simulink model "sampleModel1561_4"  (R2023a)
settings: Solver=VariableStepAuto  StartTime=0.0  StopTime=10.0  RelTol=1e-3
libraries: hdlsllib x5, simulink x2
settings Model: Creator=user1  LastModifiedBy=user1

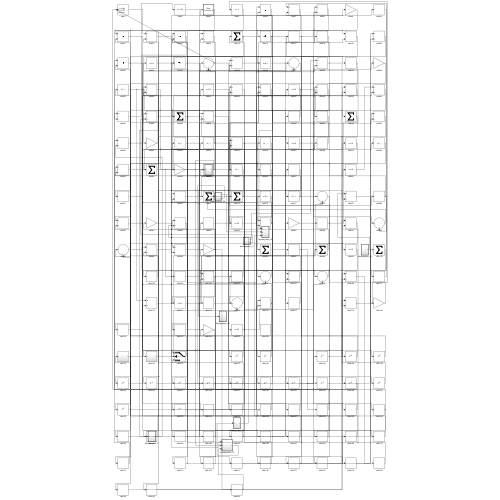
[thumbnail: Simulink's stored preview of the top-level diagram]
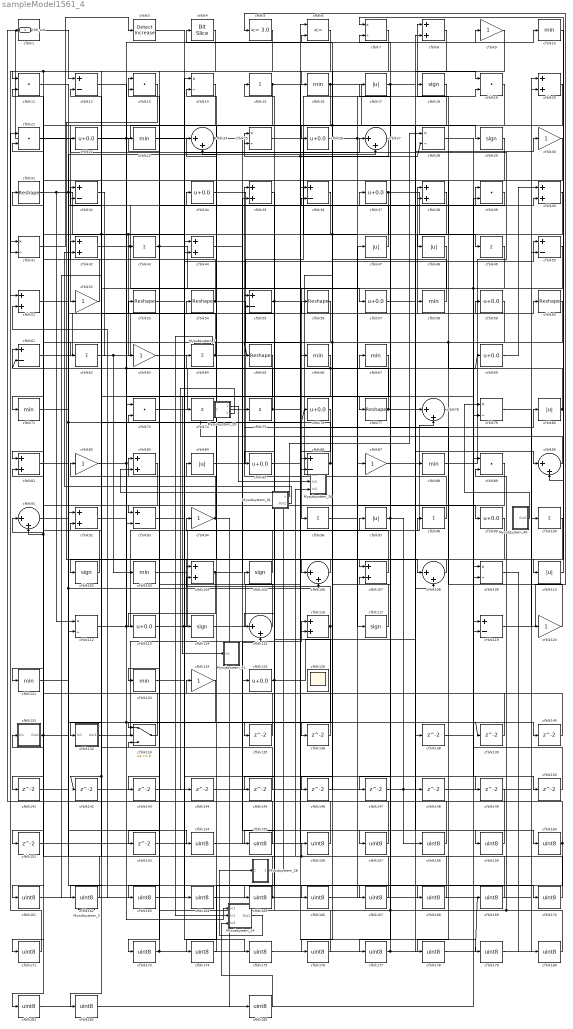
== system sampleModel1561_4 ==
  Mysubsystem_14 : Subsystem  TreatAsAtomicUnit=on  RTWFcnName=Mysubsystem_14
      settings: RTWFcnNameOpts=User specified  RTWFileNameOpts=Use function name
  Mysubsystem_26 : Subsystem  TreatAsAtomicUnit=on  RTWFcnName=Mysubsystem_26
      settings: RTWFcnNameOpts=User specified  RTWFileNameOpts=Use function name
  Mysubsystem_28 : Subsystem  TreatAsAtomicUnit=on  RTWFcnName=Mysubsystem_28
      settings: RTWFcnNameOpts=User specified  RTWFileNameOpts=Use function name
  Mysubsystem_29 : Subsystem  TreatAsAtomicUnit=on  RTWFcnName=Mysubsystem_29
      settings: RTWFcnNameOpts=User specified  RTWFileNameOpts=Use function name
  Mysubsystem_3 : Subsystem  TreatAsAtomicUnit=on  RTWFcnName=Mysubsystem_3
      settings: RTWFcnNameOpts=User specified  RTWFileNameOpts=Use function name
  Mysubsystem_31 : Subsystem  TreatAsAtomicUnit=on  RTWFcnName=Mysubsystem_31
      settings: RTWFcnNameOpts=User specified  RTWFileNameOpts=Use function name
  Mysubsystem_40 : Subsystem  TreatAsAtomicUnit=on  RTWFcnName=Mysubsystem_40
      settings: RTWFcnNameOpts=User specified  RTWFileNameOpts=Use function name
  Mysubsystem_41 : Subsystem  TreatAsAtomicUnit=on  RTWFcnName=Mysubsystem_41
      settings: RTWFcnNameOpts=User specified  RTWFileNameOpts=Use function name
  Mysubsystem_7 : Subsystem  TreatAsAtomicUnit=on  RTWFcnName=Mysubsystem_7
      settings: RTWFcnNameOpts=User specified  RTWFileNameOpts=Use function name
  cfblk1 : simulink/Logic and Bit Operations/Bit Set  iBit=0
      settings: LibrarySourceBlock=|
      | hdlsllib/Logic and Bit
      | Operations/Bit Set
  cfblk{10,16,23,58,66..67,71,88,103,121,123} (11 alike) : MinMax  OutDataTypeStr=uint8
  cfblk{15,43,49,62,64,74..75,96,98,100} (10 alike) : Sum  Inputs=+  OutDataTypeStr=uint8
  cfblk{18,29,102,105,114,117} (6 alike) : Signum
  cfblk{8,20,35,38,40,42,44,51,81,83,92,104,107,116} (14 alike) : Sum  OutDataTypeStr=uint8
  cfblk{24,27,78,90..91,106,108,115} (8 alike) : Sum  Inputs=|++  OutDataTypeStr=uint8
  cfblk{7,14,25,28,41,79,109,112} (8 alike) : Product  Inputs=*/  OutDataTypeStr=uint8  RndMeth=Zero  SaturateOnIntegerOverflow=on
  cfblk{11,13,19,21,39,73,89} (7 alike) : DotProduct  OutDataTypeStr=uint8
  cfblk{17,47..48,80,84,97,110} (7 alike) : Abs  OutDataTypeStr=uint8  SaturateOnIntegerOverflow=off
  cfblk{22,26,34,37,57,59,69,76,85,99,113,125} (12 alike) : Bias  Bias=0.0  SaturateOnIntegerOverflow=off
  cfblk{12,32,36,50,55,61,86,93,119} (9 alike) : Sum  Inputs=+-  OutDataTypeStr=uint8
  cfblk{9,30,52,63,82,87,94,120,124} (9 alike) : Gain  OutDataTypeStr=uint8
  cfblk126 : Scope
      settings: Floating=on
  cfblk131 : Subsystem
      settings: LibrarySourceBlock=|
      | hdlsllib/Ports &
      | Subsystems/Subsystem
  cfblk132 : Subsystem
      settings: LibrarySourceBlock=|
      | hdlsllib/Ports &
      | Subsystems/Subsystem
  cfblk133 : Switch  OutDataTypeStr=uint8  SaturateOnIntegerOverflow=off  InputSameDT=off
  cfblk{135..136,138..151,153} (17 alike) : Delay  SampleTime=1
  cfblk{154..171,173..182,185} (29 alike) : DataTypeConversion  OutDataTypeStr=uint8  SaturateOnIntegerOverflow=off  RndMeth=Floor
  cfblk3 : simulink/Logic and Bit Operations/Detect Increase  vinit=0.0  OutDataTypeStr=uint8
      settings: LibrarySourceBlock=|
      | hdlsllib/Logic and Bit
      | Operations/Detect
      | Increase
  cfblk{31,53..54,56,60,65,77} (7 alike) : Reshape
  cfblk4 : hdlsllib/Logic and Bit Operations/Bit Slice  lidx=7  ridx=0
  cfblk5 : hdlsllib/Logic and Bit Operations/Compare To Constant  relop=<=  const=3.0  OutDataTypeStr=uint8
  cfblk6 : RelationalOperator  Operator=<=  OutDataTypeStr=boolean  InputSameDT=off
  Hdl_out : Outport  OutDataTypeStr=uint8
  wires:
  cfblk9/1 -> cfblk16/1
  cfblk89/1 -> cfblk93/1
  cfblk15/1 -> cfblk52/1, cfblk159/1
  cfblk37/1 -> Mysubsystem_26/1(In1), Mysubsystem_3/1(In1), cfblk151/1, cfblk49/1
  cfblk48/1 -> cfblk96/1
  cfblk34/1 -> cfblk57/1
  cfblk13/1 -> cfblk108/1
  cfblk88/1 -> cfblk25/1
  cfblk47/1 -> cfblk13/1
  cfblk97/1 -> cfblk148/1, cfblk158/1, cfblk147/1
  cfblk98/1 -> cfblk35/1
  cfblk66/1 -> Mysubsystem_41/1(In1), cfblk61/2
  cfblk61/1 -> cfblk38/1
  cfblk41/1 -> cfblk3/1
  cfblk58/1 -> cfblk4/1
  cfblk105/1 -> cfblk94/1
  cfblk17/1 -> cfblk77/1, cfblk19/1
  cfblk113/1 -> cfblk97/1, cfblk149/1
  cfblk64/1 -> cfblk56/1, cfblk32/1
  cfblk109/1 -> cfblk180/1
  cfblk87/1 -> cfblk160/1
  cfblk110/1 -> cfblk7/1
  cfblk62/1 -> cfblk54/1, cfblk103/1
  cfblk59/1 -> cfblk106/1, cfblk141/1
  cfblk65/1 -> cfblk142/1, cfblk182/1
  cfblk29/1 -> cfblk48/1
  cfblk99/1 -> cfblk114/1
  cfblk31/1 -> cfblk43/1, cfblk74/1, cfblk135/1, cfblk112/1
  cfblk86/1 -> cfblk32/2, cfblk136/1
  cfblk119/1 -> cfblk5/1
  cfblk69/1 -> cfblk40/1
  cfblk103/1 -> cfblk35/2
  cfblk112/1 -> cfblk69/1, cfblk55/2, cfblk78/2
  cfblk114/1 -> cfblk80/1
  cfblk74/1 -> cfblk8/1
  cfblk84/1 -> cfblk39/1
  cfblk79/1 -> cfblk120/1
  cfblk94/1 -> cfblk82/1, cfblk185/1
  cfblk36/1 -> cfblk63/1
  cfblk18/1 -> cfblk121/1
  cfblk76/1 -> cfblk86/1
  cfblk133/1 -> cfblk91/1, cfblk91/2
  cfblk104/1 -> cfblk113/1, cfblk98/1
  cfblk120/1 -> cfblk75/1
  cfblk115/1 -> cfblk83/1
  cfblk93/1 -> cfblk27/1
  cfblk80/1 -> cfblk18/1, cfblk90/2
  cfblk106/1 -> cfblk102/1
  cfblk116/1 -> cfblk104/2, cfblk163/1
  cfblk10/1 -> cfblk110/1
  cfblk25/1 -> cfblk117/1
  cfblk22/1 -> Mysubsystem_14/1(In1), cfblk29/1
  cfblk132/1(Out1) -> cfblk116/1
  cfblk107/1 -> cfblk64/1
  cfblk67/1 -> cfblk115/1
  cfblk124/1 -> cfblk173/1
  cfblk5/1 -> cfblk132/1(In1)
  cfblk92/1 -> cfblk167/1
  cfblk39/1 -> cfblk36/2
  cfblk63/1 -> cfblk50/1
  cfblk38/1 -> cfblk123/1
  cfblk75/1 -> cfblk53/1, cfblk179/1
  cfblk60/1 -> cfblk65/1, cfblk178/1
  cfblk54/1 -> cfblk66/1, cfblk11/2
  cfblk121/1 -> cfblk27/2
  cfblk20/1 -> cfblk177/1
  cfblk7/1 -> cfblk11/1
  cfblk43/1 -> cfblk125/1, cfblk153/1
  cfblk125/1 -> cfblk15/1, cfblk8/2
  cfblk42/1 -> cfblk86/2, cfblk37/1
  cfblk26/1 -> cfblk99/1, cfblk19/2
  cfblk96/1 -> cfblk58/1
  cfblk8/1 -> cfblk26/1
  cfblk77/1 -> cfblk30/1, cfblk55/1
  cfblk71/1 -> cfblk34/1
  cfblk19/1 -> cfblk104/1, cfblk146/1
  cfblk55/1 -> cfblk38/2, cfblk145/1
  cfblk85/1 -> cfblk10/1, cfblk28/2
  cfblk27/1 -> cfblk25/2
  cfblk81/1 -> cfblk76/1, cfblk60/1
  cfblk16/1 -> cfblk88/1, cfblk133/1
  cfblk100/1 -> cfblk165/1
  cfblk108/1 -> cfblk107/1
  cfblk117/1 -> cfblk22/1
  cfblk35/1 -> cfblk85/1
  cfblk50/1 -> cfblk119/2, cfblk62/1
  cfblk52/1 -> cfblk42/1
  cfblk82/1 -> cfblk93/2, cfblk9/1
  cfblk91/1 -> cfblk59/1
  cfblk123/1 -> cfblk44/1
  cfblk6/1 -> cfblk81/1, cfblk41/2
  cfblk11/1 -> cfblk133/2, cfblk139/1, cfblk106/2
  cfblk30/1 -> cfblk71/1
  cfblk12/1 -> cfblk79/2
  cfblk57/1 -> cfblk90/1
  cfblk73/1 -> cfblk67/1
  cfblk3/1 -> cfblk44/2
  cfblk131/1(Out1) -> cfblk40/2, cfblk181/1
  cfblk1/1 -> cfblk12/1
  cfblk102/1 -> cfblk61/1
  cfblk135/1 -> cfblk13/2
  cfblk136/1 -> cfblk73/1
  cfblk138/1 -> cfblk39/2
  cfblk139/1 -> cfblk107/2
  cfblk44/1 -> cfblk140/1
  cfblk140/1 -> cfblk81/2
  cfblk141/1 -> cfblk112/2
  cfblk142/1 -> cfblk78/1
  cfblk4/1 -> cfblk143/1
  cfblk144/1 -> cfblk36/1
  cfblk145/1 -> cfblk12/2
  cfblk146/1 -> cfblk6/2
  cfblk147/1 -> cfblk108/2
  cfblk148/1 -> cfblk50/2
  cfblk149/1 -> cfblk1/1
  cfblk28/1 -> cfblk150/1
  cfblk150/1 -> cfblk119/1
  cfblk151/1 -> cfblk116/2
  cfblk153/1 -> cfblk115/2
  cfblk21/1 -> cfblk154/1
  cfblk154/1 -> cfblk6/1
  cfblk49/1 -> cfblk155/1
  cfblk155/1 -> cfblk21/1
  cfblk156/1 -> cfblk21/2
  cfblk24/1 -> cfblk157/1, Hdl_out/1
  cfblk157/1 -> cfblk41/1
  cfblk158/1 -> cfblk24/1
  cfblk159/1 -> cfblk24/2
  cfblk160/1 -> cfblk133/3, cfblk174/1
  cfblk56/1 -> cfblk161/1
  cfblk161/1 -> cfblk87/1
  cfblk14/1 -> cfblk162/1
  cfblk162/1 -> cfblk31/1
  cfblk163/1 -> cfblk14/1
  cfblk143/1 -> cfblk164/1
  cfblk164/1 -> cfblk14/2
  cfblk165/1 -> cfblk131/1(In1), cfblk47/1
  cfblk53/1 -> cfblk166/1
  cfblk166/1 -> cfblk100/1
  cfblk167/1 -> Mysubsystem_26/3(In3), cfblk156/1
  cfblk78/1 -> cfblk168/1
  cfblk168/1 -> cfblk92/1
  cfblk169/1 -> cfblk92/2
  cfblk51/1 -> cfblk170/1
  cfblk170/1 -> cfblk84/1
  cfblk83/1 -> cfblk171/1
  cfblk171/1 -> cfblk51/1
  cfblk173/1 -> cfblk169/1, cfblk73/2
  cfblk174/1 -> cfblk124/1
  cfblk23/1 -> cfblk175/1
  cfblk175/1 -> cfblk89/1
  cfblk40/1 -> cfblk176/1
  cfblk176/1 -> cfblk23/1
  cfblk177/1 -> cfblk138/1, cfblk7/2
  cfblk178/1 -> cfblk20/1
  cfblk179/1 -> cfblk20/2
  cfblk180/1 -> cfblk17/1, cfblk105/1, cfblk89/2
  cfblk181/1 -> cfblk109/1
  cfblk182/1 -> cfblk109/2
  Mysubsystem_3/1(Out1) -> cfblk51/2
  cfblk32/1 -> Mysubsystem_7/1(u)
  Mysubsystem_7/1(Out1) -> Mysubsystem_14/2(In2)
  cfblk185/1 -> Mysubsystem_14/3(In3)
  Mysubsystem_14/1(Out1) -> Mysubsystem_28/1(In1)
  Mysubsystem_28/1(Out1) -> cfblk83/2
  cfblk90/1 -> Mysubsystem_29/1(In1)
  Mysubsystem_29/1(Out1) -> Mysubsystem_26/2(In2)
  Mysubsystem_29/2(Out2) -> cfblk144/1
  Mysubsystem_31/1(y) -> cfblk28/1
  Mysubsystem_31/2(Out2) -> cfblk42/2
  Mysubsystem_40/1(Out1) -> cfblk79/1

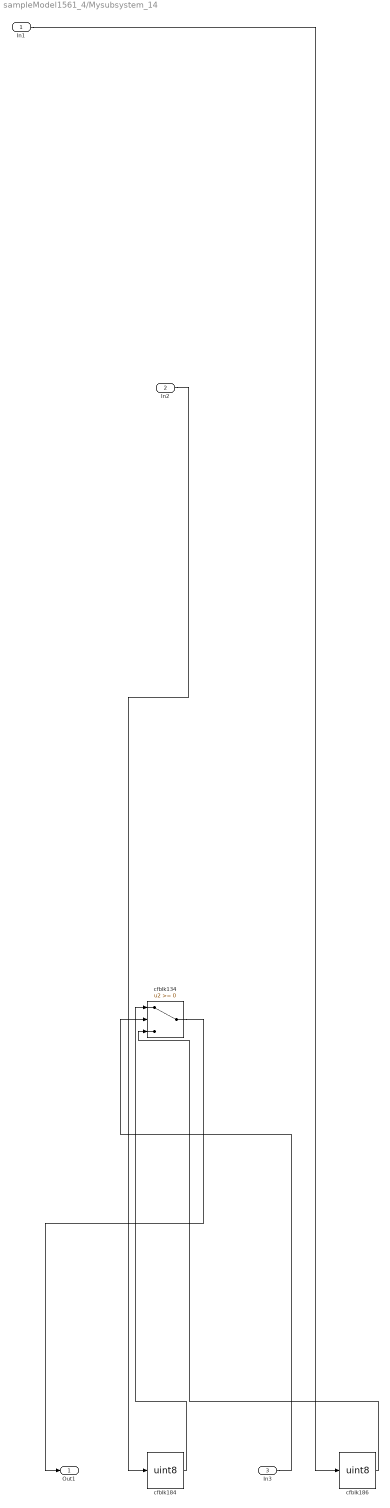
== system sampleModel1561_4/Mysubsystem_14 ==
  In1 : Inport
  In2 : Inport  Port=2
  In3 : Inport  Port=3
  cfblk134 : Switch  SaturateOnIntegerOverflow=off  InputSameDT=off
  cfblk184 : DataTypeConversion  OutDataTypeStr=uint8  SaturateOnIntegerOverflow=off  RndMeth=Floor
  cfblk186 : DataTypeConversion  OutDataTypeStr=uint8  SaturateOnIntegerOverflow=off  RndMeth=Floor
  Out1 : Outport
  wires:
  cfblk134/1 -> Out1/1
  cfblk186/1 -> cfblk134/3
  cfblk184/1 -> cfblk134/1
  In2/1 -> cfblk184/1
  In1/1 -> cfblk186/1
  In3/1 -> cfblk134/2

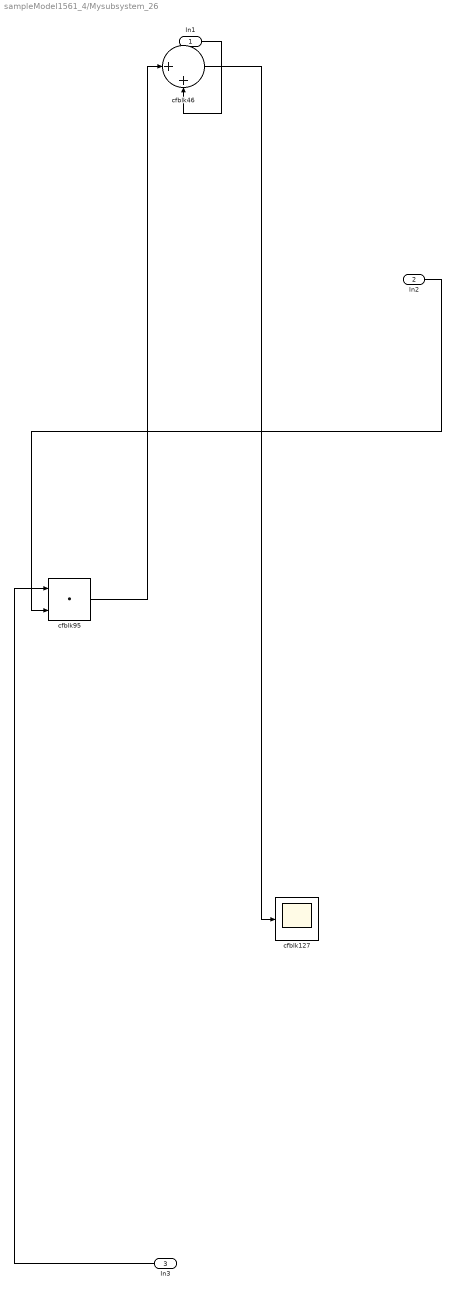
== system sampleModel1561_4/Mysubsystem_26 ==
  In1 : Inport
  In2 : Inport  Port=2
  In3 : Inport  Port=3
  cfblk127 : Scope
  cfblk46 : Sum  Inputs=|++
  cfblk95 : DotProduct  OutDataTypeStr=Inherit: Inherit via internal rule
  wires:
  cfblk95/1 -> cfblk46/1
  In1/1 -> cfblk46/2
  cfblk46/1 -> cfblk127/1
  In2/1 -> cfblk95/2
  In3/1 -> cfblk95/1

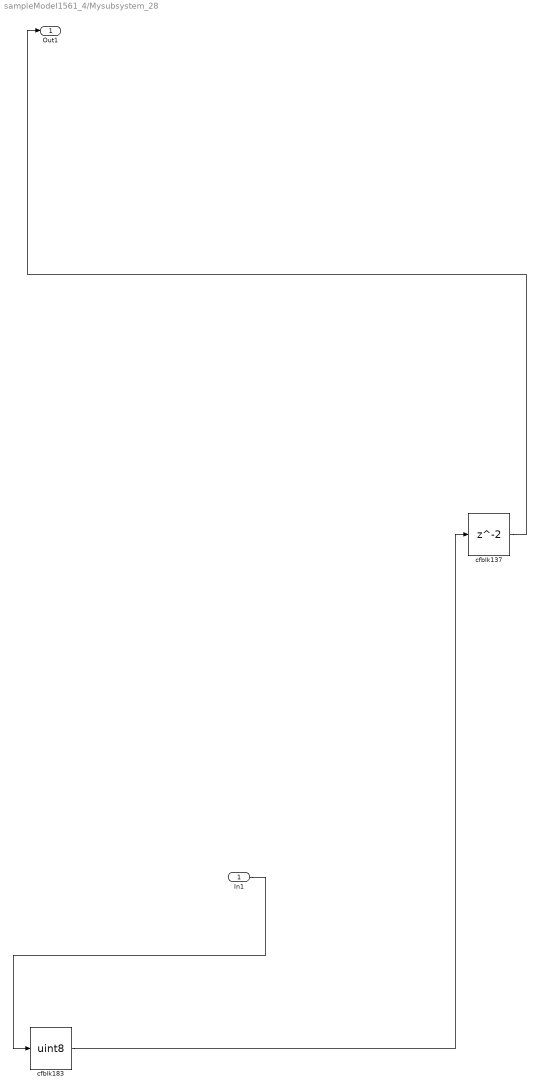
== system sampleModel1561_4/Mysubsystem_28 ==
  In1 : Inport
  cfblk137 : Delay  SampleTime=1
  cfblk183 : DataTypeConversion  OutDataTypeStr=uint8  SaturateOnIntegerOverflow=off  RndMeth=Floor
  Out1 : Outport
  wires:
  cfblk183/1 -> cfblk137/1
  cfblk137/1 -> Out1/1
  In1/1 -> cfblk183/1

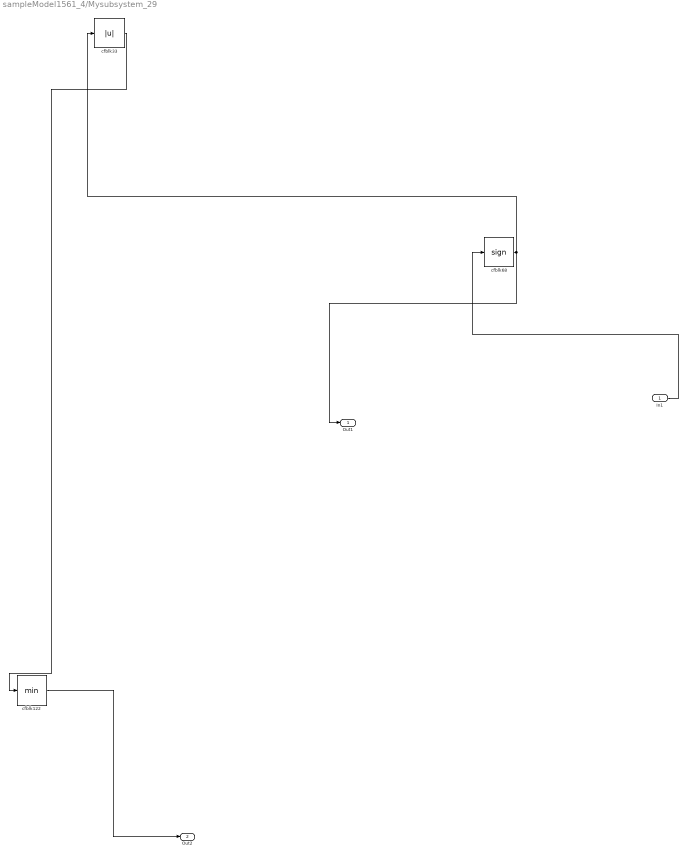
== system sampleModel1561_4/Mysubsystem_29 ==
  In1 : Inport
  cfblk122 : MinMax
  cfblk33 : Abs  SaturateOnIntegerOverflow=off
  cfblk68 : Signum
  Out1 : Outport
  Out2 : Outport  Port=2
  wires:
  cfblk33/1 -> cfblk122/1
  cfblk68/1 -> Out1/1, cfblk33/1
  cfblk122/1 -> Out2/1
  In1/1 -> cfblk68/1

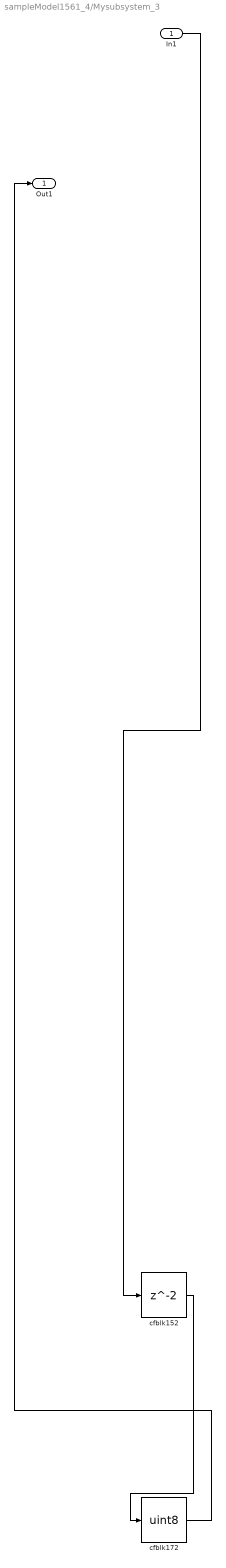
== system sampleModel1561_4/Mysubsystem_3 ==
  In1 : Inport
  cfblk152 : Delay  SampleTime=1
  cfblk172 : DataTypeConversion  OutDataTypeStr=uint8  SaturateOnIntegerOverflow=off  RndMeth=Floor
  Out1 : Outport
  wires:
  cfblk172/1 -> Out1/1
  In1/1 -> cfblk152/1
  cfblk152/1 -> cfblk172/1

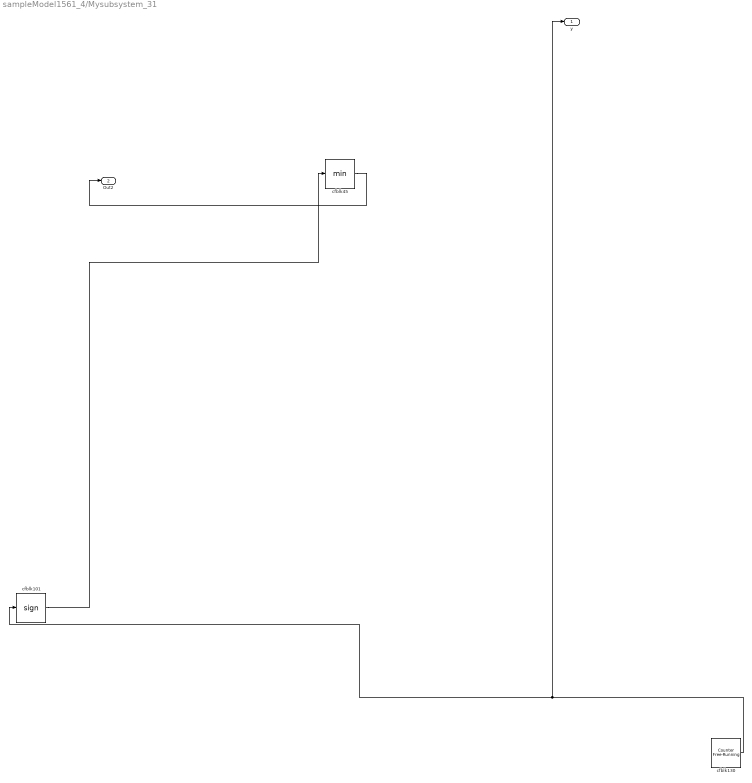
== system sampleModel1561_4/Mysubsystem_31 ==
  cfblk101 : Signum
  cfblk130 : hdlsllib/Sources/Counter Free-Running  NumBits=16  tsamp=-1
  cfblk45 : MinMax
  y : Outport
  Out2 : Outport  Port=2
  wires:
  cfblk101/1 -> cfblk45/1
  cfblk130/1 -> y/1, cfblk101/1
  cfblk45/1 -> Out2/1

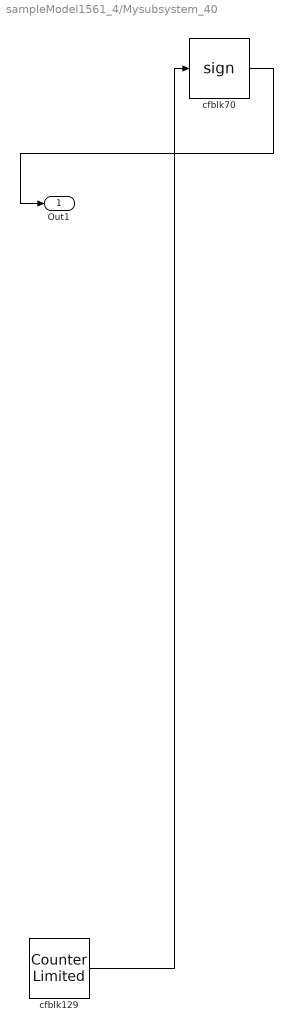
== system sampleModel1561_4/Mysubsystem_40 ==
  cfblk129 : hdlsllib/Sources/Counter Limited  uplimit=7  tsamp=-1
  cfblk70 : Signum
  Out1 : Outport
  wires:
  cfblk129/1 -> cfblk70/1
  cfblk70/1 -> Out1/1

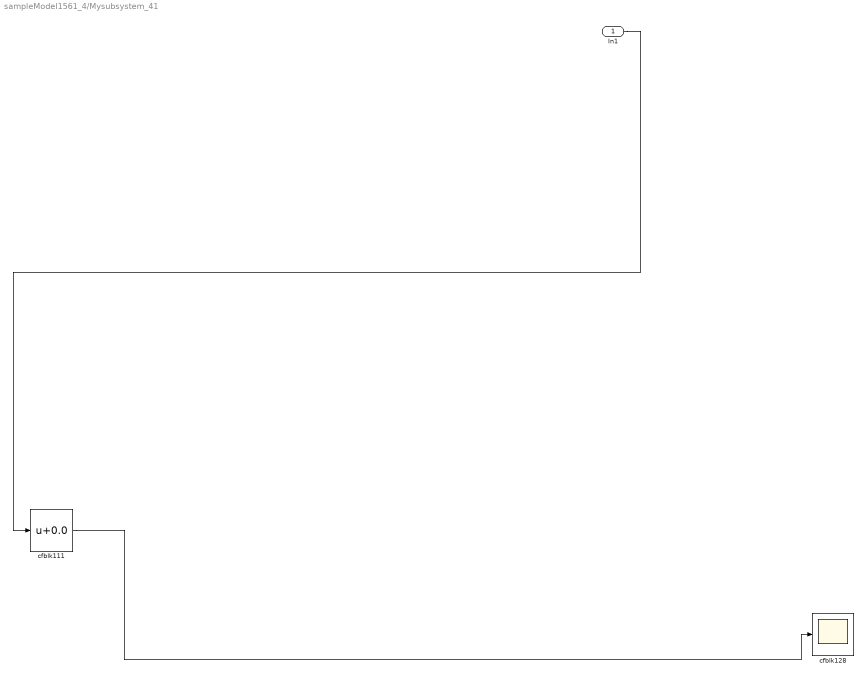
== system sampleModel1561_4/Mysubsystem_41 ==
  In1 : Inport
  cfblk111 : Bias  Bias=0.0  SaturateOnIntegerOverflow=off
  cfblk128 : Scope
  wires:
  cfblk111/1 -> cfblk128/1
  In1/1 -> cfblk111/1

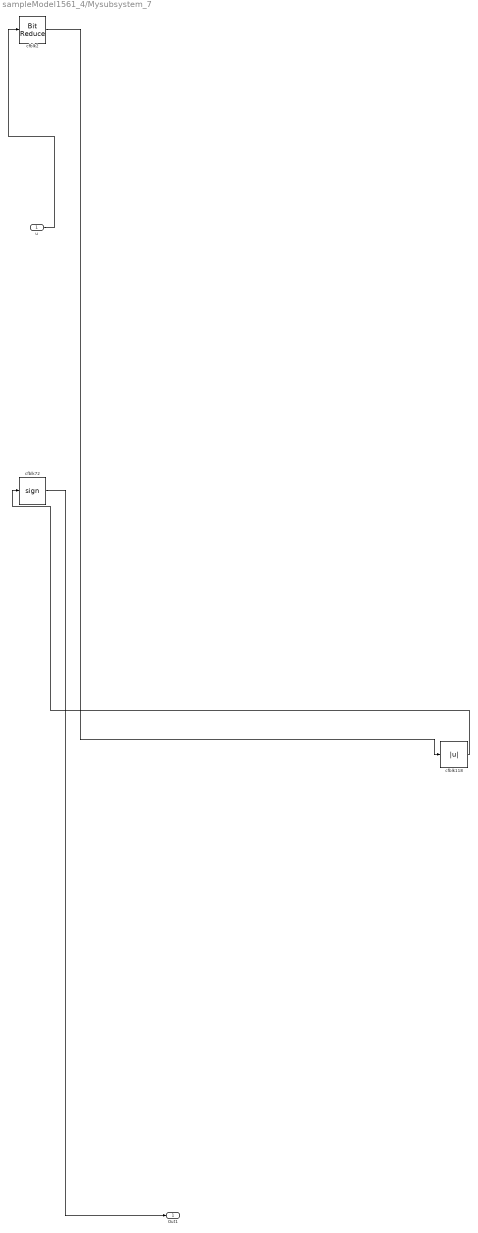
== system sampleModel1561_4/Mysubsystem_7 ==
  u : Inport
  cfblk118 : Abs  SaturateOnIntegerOverflow=off
  cfblk2 : hdlsllib/Logic and Bit Operations/Bit Reduce  mode=AND
  cfblk72 : Signum
  Out1 : Outport
  wires:
  u/1 -> cfblk2/1
  cfblk2/1 -> cfblk118/1
  cfblk118/1 -> cfblk72/1
  cfblk72/1 -> Out1/1

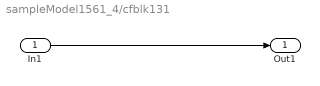
== system sampleModel1561_4/cfblk131 ==
  In1 : Inport
  Out1 : Outport
  wires:
  In1/1 -> Out1/1

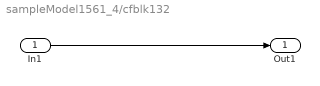
== system sampleModel1561_4/cfblk132 ==
  In1 : Inport
  Out1 : Outport
  wires:
  In1/1 -> Out1/1
